simulink model "circuitbd"  (R2015a)
settings: Solver=ode45  StartTime=0.0  StopTime=10.0  RelTol=1e-3
undefined symbols (not defined in the file): Cap, L, R
settings Model: Creator=eechris  LastModifiedBy=eechris
settings DataIOCC: SignalLoggingSaveFormat=ModelDataLogs
settings OptimizationCC: ExpressionDepthLimit=2147483647
settings DebuggingCC: UnderspecifiedInitializationDetection=Classic  MergeDetectMultiDrivingBlocksExec=none  SolverPrmCheckMsg=warning  FcnCallInpInsideContextMsg=UseLocalSettings  StateNameClashWarn=warning  StrictBusMsg=Warning
settings GRTTargetCC: CombineOutputUpdateFcns=off  GRTInterface=on

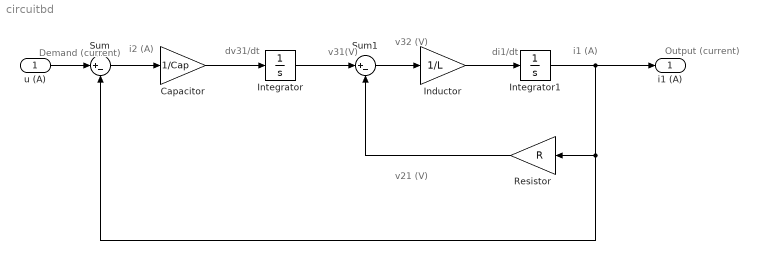
== system circuitbd ==
  note: i2 (A)
  note: dv31/dt
  note: v31(V)
  note: v32 (V)
  note: di1/dt
  note: i1 (A)
  note: v21 (V)
  note: Demand (current)
  note: Output (current)
  u (A) : Inport
  Capacitor : Gain  Gain=1/Cap
  Inductor : Gain  Gain=1/L
  Integrator : Integrator
  Integrator1 : Integrator
  Resistor : Gain  Gain=R
  Sum : Sum  Inputs=|+-
  Sum1 : Sum  Inputs=|+-
  i1 (A) : Outport
  wires:
  u (A)/1 -> Sum/1
  Sum/1 -> Capacitor/1
  Capacitor/1 -> Integrator/1
  Integrator/1 -> Sum1/1
  Sum1/1 -> Inductor/1
  Inductor/1 -> Integrator1/1
  Resistor/1 -> Sum1/2
  Integrator1/1 -> Resistor/1, Sum/2, i1 (A)/1
